simulink model "apsfsm_torque_compensation_wrapper"  (R2026a)
settings: Solver=FixedStepDiscrete  StopTime=0.01  FixedStep=5e-4
settings Model: Creator=ASUS  LastModifiedBy=ASUS
settings HardwareCC: ProdLargestAtomicInteger=Long  ProdLargestAtomicFloat=Double  ProdHWDeviceType=ARM Compatible->ARM Cortex
settings RTWCC: SystemTargetFile=ert.tlc  GenCodeOnly=on  Description=Embedded Coder
settings CodeAppCC: MaxIdLength=63.0

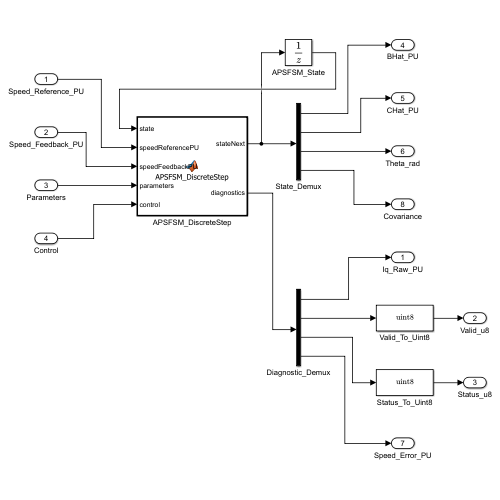
[thumbnail: Simulink's stored preview of the top-level diagram]
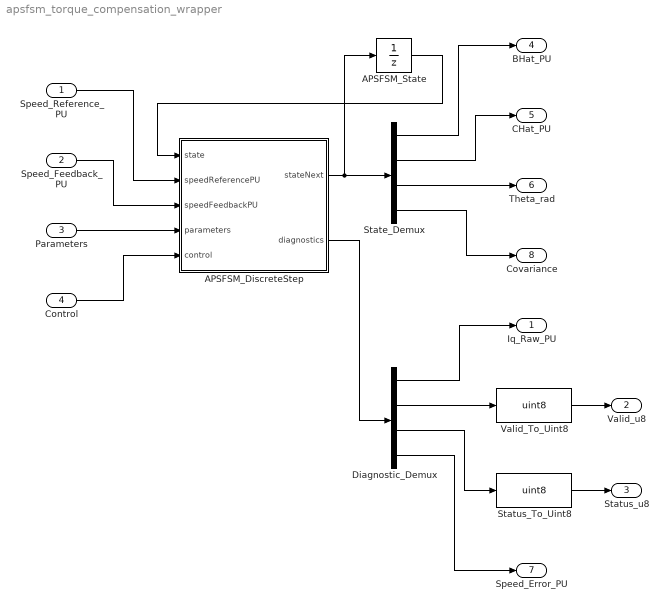
== system apsfsm_torque_compensation_wrapper ==
  Speed_Reference_PU : Inport  OutDataTypeStr=single  PortDimensions=1
  Speed_Feedback_PU : Inport  Port=2  OutDataTypeStr=single  PortDimensions=1
  Parameters : Inport  Port=3  OutDataTypeStr=single  PortDimensions=5
  Control : Inport  Port=4  OutDataTypeStr=single  PortDimensions=3
  APSFSM_DiscreteStep : MATLAB Function  TreatAsAtomicUnit=on
  APSFSM_State : UnitDelay  InitialCondition=single([0;0;0;0])  SampleTime=-1
  Diagnostic_Demux : Demux
  State_Demux : Demux
  Status_To_Uint8 : DataTypeConversion  OutDataTypeStr=uint8
  Valid_To_Uint8 : DataTypeConversion  OutDataTypeStr=uint8
  Iq_Raw_PU : Outport  OutDataTypeStr=single
  Valid_u8 : Outport  Port=2  OutDataTypeStr=uint8
  Status_u8 : Outport  Port=3  OutDataTypeStr=uint8
  BHat_PU : Outport  Port=4  OutDataTypeStr=single
  CHat_PU : Outport  Port=5  OutDataTypeStr=single
  Theta_rad : Outport  Port=6  OutDataTypeStr=single
  Speed_Error_PU : Outport  Port=7  OutDataTypeStr=single
  Covariance : Outport  Port=8  OutDataTypeStr=single
  wires:
  APSFSM_State/1 -> APSFSM_DiscreteStep/1(state)
  Speed_Reference_PU/1 -> APSFSM_DiscreteStep/2(speedReferencePU)
  Speed_Feedback_PU/1 -> APSFSM_DiscreteStep/3(speedFeedbackPU)
  Parameters/1 -> APSFSM_DiscreteStep/4(parameters)
  Control/1 -> APSFSM_DiscreteStep/5(control)
  APSFSM_DiscreteStep/1(stateNext) -> State_Demux/1, APSFSM_State/1
  APSFSM_DiscreteStep/2(diagnostics) -> Diagnostic_Demux/1
  Diagnostic_Demux/1 -> Iq_Raw_PU/1
  Diagnostic_Demux/2 -> Valid_To_Uint8/1
  Valid_To_Uint8/1 -> Valid_u8/1
  Diagnostic_Demux/3 -> Status_To_Uint8/1
  Status_To_Uint8/1 -> Status_u8/1
  State_Demux/1 -> BHat_PU/1
  State_Demux/2 -> CHat_PU/1
  State_Demux/3 -> Theta_rad/1
  Diagnostic_Demux/4 -> Speed_Error_PU/1
  State_Demux/4 -> Covariance/1

== matlab function apsfsm_torque_compensation_wrapper/APSFSM_DiscreteStep ==
  data: state input; stateNext output; speedReferencePU input; speedFeedbackPU input; parameters input; control input; diagnostics output
function [stateNext, diagnostics] = APSFSM_DiscreteStep(state, speedReferencePU, speedFeedbackPU, parameters, control)
%#codegen
[stateNext, diagnostics] = apsfsmTorqueCompensationStep(state, speedReferencePU, speedFeedbackPU, parameters, control);
end
